simulink model "DCMotorModel"  (R2023b)
settings: Solver=VariableStepAuto  StartTime=0.0  StopTime=10.0  RelTol=1e-3
values from neighbouring files (symbols this model uses):
  Kb = 0.125    [DCModel.m]
  Kma = 0.127    [DCModel.m]
  Tl = 20    [DCModel.m]
  Va = 20    [DCModel.m]
undefined symbols (not defined in the file or in its folder): denTF, denTF1, numTF, numTF1
settings Model: Creator=CHIBIK  LastModifiedBy=CHIBIK

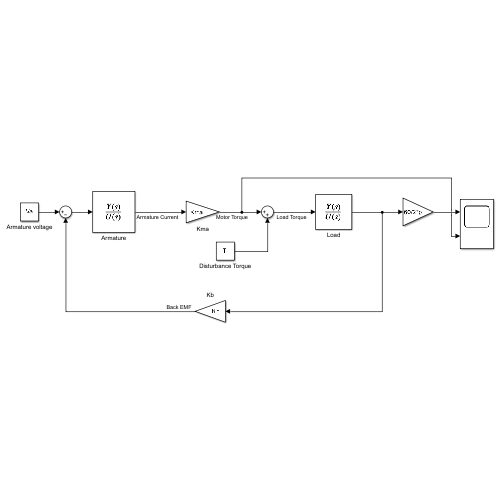
[thumbnail: Simulink's stored preview of the top-level diagram]
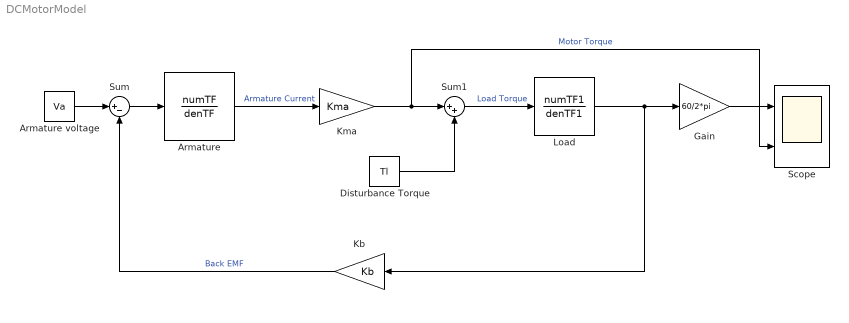
== system DCMotorModel ==
  Armature : TransferFcn  Numerator=numTF  Denominator=denTF
  Armature voltage : Constant  Value=Va
  Disturbance Torque : Constant  Value=Tl
  Gain : Gain  Gain=60/2*pi
  Kb : Gain  Gain=Kb
  Kma : Gain  Gain=Kma
  Load : TransferFcn  Numerator=numTF1  Denominator=denTF1
  Scope : Scope  NumInputPorts=2
  Sum : Sum  Inputs=|+-
  Sum1 : Sum  Inputs=|++
  wires:
  Armature voltage/1 -> Sum/1
  Sum/1 -> Armature/1
  Armature/1 -> Kma/1  "Armature Current"
  Kma/1 -> Scope/2, Sum1/1  "Motor Torque"
  Sum1/1 -> Load/1  "Load Torque"
  Disturbance Torque/1 -> Sum1/2
  Load/1 -> Kb/1, Gain/1
  Kb/1 -> Sum/2  "Back EMF"
  Gain/1 -> Scope/1
